simulink model "FCS_MPC_6ph_Regelungsmodell"  (R2022a)
settings: Solver=ode23t  StartTime=0.0  StopTime=0.1  RelTol=1e-3  AbsTol=1e-3  EnableMultiTasking=on
values from neighbouring files (symbols this model uses):
  f_c = 100000    [Params_testbench.m]
  L_d = 0.0001473    [Params_testbench.m]
  L_q = 0.0001484    [Params_testbench.m]
  L_x = 0.00005566    (= 5.566e-05)    [Params_testbench.m]
  L_y = L_x    (= 5.566e-05)    [Params_testbench.m]
  p = 5    [Params_testbench.m]
  psi_pm = 0.0048    [Params_testbench.m]
  R_ph = 0.1278    [Params_testbench.m]
  T_100MHz = 1/f_100MHz    (= 1e-08)    [Params_testbench.m]
  u_dc = 36.0    (= 36)    [Params_testbench.m]
libraries: hdlsllib x53, nesl_utility x39, fl_lib x32, ee_lib x12, simulink x8, spsAlphaBetaZerotodq0Lib x1
(part 5 of 8)

== system FCS_MPC_6ph_Regelungsmodell/Microcontroller Software/Switching_states ==
  I : Inport
  valid_in : Inport  Port=2
  Delay{,1..15} (16 alike) : Delay  DelayLength=1
  Demux : Demux  Outputs=12
  Detect Rise Positive : hdlsllib/Logic and Bit Operations/Detect Rise Positive  vinit=0  OutDataTypeStr=boolean
      settings: SourceProductBaseCode=SL
  MATLAB Function1 : MATLAB Function  TreatAsAtomicUnit=on
  Switch_on2 : Switch  Threshold=1  OutDataTypeStr=Inherit: Inherit via back propagation  RndMeth=Simplest  SaturateOnIntegerOverflow=off  InputSameDT=off
  HB1T : Outport
  HB1B : Outport  Port=2
  HB2T : Outport  Port=3
  HB2B : Outport  Port=4
  HB3T : Outport  Port=5
  HB3B : Outport  Port=6
  HB4T : Outport  Port=7
  HB4B : Outport  Port=8
  HB5T : Outport  Port=9
  HB5B : Outport  Port=10
  HB6T : Outport  Port=11
  HB6B : Outport  Port=12
  done : Outport  Port=13
  wires:
  Demux/4 -> Delay12/1
  I/1 -> Delay1/1
  Demux/6 -> Delay10/1
  Demux/12 -> Delay4/1
  Switch_on2/1 -> MATLAB Function1/1(I), Delay2/1
  Demux/8 -> Delay8/1
  valid_in/1 -> Delay/1
  Demux/7 -> Delay9/1
  Demux/2 -> Delay14/1
  Detect Rise Positive/1 -> Delay3/1, Switch_on2/2  "End_Cycle"
  Demux/5 -> Delay11/1
  Delay2/1 -> Switch_on2/3
  Demux/1 -> Delay15/1
  Demux/9 -> Delay7/1
  Demux/10 -> Delay6/1
  MATLAB Function1/1(next_switching_state) -> Demux/1
  Demux/3 -> Delay13/1
  Delay/1 -> Detect Rise Positive/1
  Delay1/1 -> Switch_on2/1
  Delay3/1 -> done/1
  Delay4/1 -> HB6B/1
  Demux/11 -> Delay5/1
  Delay5/1 -> HB6T/1
  Delay6/1 -> HB5B/1
  Delay7/1 -> HB5T/1
  Delay8/1 -> HB4B/1
  Delay9/1 -> HB4T/1
  Delay10/1 -> HB3B/1
  Delay11/1 -> HB3T/1
  Delay12/1 -> HB2B/1
  Delay13/1 -> HB2T/1
  Delay14/1 -> HB1B/1
  Delay15/1 -> HB1T/1

== system FCS_MPC_6ph_Regelungsmodell/Microcontroller Software/Switching_states1 ==
  I : Inport
  valid_in : Inport  Port=2
  Delay{,1..15} (16 alike) : Delay  DelayLength=1
  Demux : Demux  Outputs=12
  Detect Rise Positive : hdlsllib/Logic and Bit Operations/Detect Rise Positive  vinit=0  OutDataTypeStr=boolean
      settings: SourceProductBaseCode=SL
  MATLAB Function1 : MATLAB Function  TreatAsAtomicUnit=on
  Switch_on2 : Switch  Threshold=1  OutDataTypeStr=Inherit: Inherit via back propagation  RndMeth=Simplest  SaturateOnIntegerOverflow=off  InputSameDT=off
  HB1T : Outport
  HB1B : Outport  Port=2
  HB2T : Outport  Port=3
  HB2B : Outport  Port=4
  HB3T : Outport  Port=5
  HB3B : Outport  Port=6
  HB4T : Outport  Port=7
  HB4B : Outport  Port=8
  HB5T : Outport  Port=9
  HB5B : Outport  Port=10
  HB6T : Outport  Port=11
  HB6B : Outport  Port=12
  done : Outport  Port=13
  wires:
  Demux/4 -> Delay12/1
  I/1 -> Delay1/1
  Demux/6 -> Delay10/1
  Demux/12 -> Delay4/1
  Switch_on2/1 -> MATLAB Function1/1(I), Delay2/1
  Demux/8 -> Delay8/1
  valid_in/1 -> Delay/1
  Demux/7 -> Delay9/1
  Demux/2 -> Delay14/1
  Detect Rise Positive/1 -> Delay3/1, Switch_on2/2  "End_Cycle"
  Demux/5 -> Delay11/1
  Delay2/1 -> Switch_on2/3
  Demux/1 -> Delay15/1
  Demux/9 -> Delay7/1
  Demux/10 -> Delay6/1
  MATLAB Function1/1(next_switching_state) -> Demux/1
  Demux/3 -> Delay13/1
  Delay/1 -> Detect Rise Positive/1
  Delay1/1 -> Switch_on2/1
  Delay3/1 -> done/1
  Delay4/1 -> HB6B/1
  Demux/11 -> Delay5/1
  Delay5/1 -> HB6T/1
  Delay6/1 -> HB5B/1
  Delay7/1 -> HB5T/1
  Delay8/1 -> HB4B/1
  Delay9/1 -> HB4T/1
  Delay10/1 -> HB3B/1
  Delay11/1 -> HB3T/1
  Delay12/1 -> HB2B/1
  Delay13/1 -> HB2T/1
  Delay14/1 -> HB1B/1
  Delay15/1 -> HB1T/1

== system FCS_MPC_6ph_Regelungsmodell/Microcontroller Software/vsd_and_park_tra ==
  i_a1 : Inport
  i_b1 : Inport  Port=2
  i_c1 : Inport  Port=3
  i_a2 : Inport  Port=4
  i_b2 : Inport  Port=5
  i_c2 : Inport  Port=6
  theta_el : Inport  Port=7
  theta_el_offset_ : Inport  Port=8
  curent_valid_in : Inport  Port=9
  Add1 : Sum  Inputs=+-  OutDataTypeStr=Inherit: Same as accumulator  RndMeth=Simplest
  Add2 : Sum  Inputs=-+  RndMeth=Simplest  OutDataTypeStr=Inherit: Same as first input
  Add3 : Sum  RndMeth=Simplest  OutDataTypeStr=Inherit: Same as first input
  Compare To Constant : hdlsllib/Logic and Bit Operations/Compare To Constant  relop=>=  const=2*pi  OutDataTypeStr=boolean
      settings: SourceProductBaseCode=SL
  Compare To Constant1 : hdlsllib/Logic and Bit Operations/Compare To Constant  relop=<  const=0  OutDataTypeStr=boolean
      settings: SourceProductBaseCode=SL
  Constant : Constant  Value=2*pi  OutDataTypeStr=single  SampleTime=1.0000e-08
  Constant1 : Constant  Value=2*pi  OutDataTypeStr=single  SampleTime=1.0000e-08
  Delay{1..6,8,25} (8 alike) : Delay  DelayLength=1
  Detect Rise Positive : hdlsllib/Logic and Bit Operations/Detect Rise Positive  vinit=0  OutDataTypeStr=boolean
      settings: SourceProductBaseCode=SL
  Gain : Gain  Commented=on  Gain=2*pi  OutDataTypeStr=Inherit: Same as input  ParamDataTypeStr=Inherit: Same as input
  MATLAB Function : MATLAB Function  TreatAsAtomicUnit=on
  MATLAB Function1 : MATLAB Function  Commented=on  TreatAsAtomicUnit=on
  Sincos : Trigonometry  Operator=sincos
  Sine HDL Optimized : hdlsllib/Lookup Tables/Cosine HDL Optimized  Commented=on  OutputFormula=sin(2*pi*u) and cos(2*pi*u)  NumDataPoints=512  TableDataTypeStr=fixdt(1,17,11)  SimulateLUTROMDelay=off
      settings: SourceProductBaseCode=SL
  Switch : Switch  Criteria=u2 > Threshold  RndMeth=Simplest  SaturateOnIntegerOverflow=off  InputSameDT=off  OutDataTypeStr=Inherit: Same as first input
  Switch1 : Switch  Criteria=u2 > Threshold  RndMeth=Simplest  SaturateOnIntegerOverflow=off  InputSameDT=off  OutDataTypeStr=Inherit: Same as first input
  Switch_on{1..8} (8 alike) : Switch  Threshold=1  RndMeth=Simplest  SaturateOnIntegerOverflow=off  InputSameDT=off  OutDataTypeStr=Inherit: Same as first input
  i_alpha : Outport
  i_alpha_axi : Outport  Port=2
  i_beta : Outport  Port=3
  i_beta_axi : Outport  Port=4
  i_d : Outport  Port=5
  i_d_axi : Outport  Port=6
  i_q : Outport  Port=7
  i_q_axi : Outport  Port=8
  i_x : Outport  Port=9
  i_x_axi : Outport  Port=10
  i_y : Outport  Port=11
  i_y_axi : Outport  Port=12
  i_0_plus : Outport  Port=13
  i_0_plus_axi : Outport  Port=14
  i_0_minus : Outport  Port=15
  i_0_minus_axi : Outport  Port=16
  done : Outport  Port=17
  i_a1_axi : Outport  Port=18
  i_b1_axi : Outport  Port=19
  i_c1_axi : Outport  Port=20
  i_a2_axi : Outport  Port=21
  i_b2_axi : Outport  Port=22
  i_c2_axi : Outport  Port=23
  theta_test : Outport  Port=24
  wires:
  i_c2/1 -> Switch_on5/1  "End_Cycle"
  Switch_on8/1 -> Add1/1, Delay8/1
  Delay8/1 -> Switch_on8/3
  Detect Rise Positive/1 -> done/1, Switch_on7/2, Switch_on6/2, Switch_on1/2, Switch_on2/2, Switch_on3/2, Switch_on4/2, Switch_on5/2, Switch_on8/2  "End_Cycle"
  Delay4/1 -> Switch_on4/3
  Switch_on2/1 -> Delay2/1, i_c1_axi/1, MATLAB Function/3(i_c1)
  Delay1/1 -> Switch_on1/3
  Switch_on1/1 -> Delay1/1, i_b1_axi/1, MATLAB Function/2(i_b1)
  Switch_on6/1 -> i_a1_axi/1, MATLAB Function/1(i_a1), Delay6/1
  Switch_on4/1 -> Delay4/1, i_b2_axi/1, MATLAB Function/5(i_b2)
  curent_valid_in/1 -> Detect Rise Positive/1  "End_Cycle"
  Switch/1 -> Switch1/3
  Switch_on3/1 -> i_a2_axi/1, MATLAB Function/4(i_a2), Delay3/1
  Delay6/1 -> Switch_on6/3
  Constant/1 -> Add2/1
  Add1/1 -> Switch/3, Compare To Constant1/1, Add3/1, Compare To Constant/1, Add2/2
  Delay2/1 -> Switch_on2/3
  Constant1/1 -> Add3/2
  theta_el/1 -> Switch_on8/1  "End_Cycle"
  Delay3/1 -> Switch_on3/3
  i_a1/1 -> Switch_on6/1  "End_Cycle"
  i_b2/1 -> Switch_on4/1  "End_Cycle"
  Add2/1 -> Switch/1
  i_a2/1 -> Switch_on3/1  "End_Cycle"
  i_b1/1 -> Switch_on1/1  "End_Cycle"
  Delay5/1 -> Switch_on5/3
  Add3/1 -> Switch1/1
  i_c1/1 -> Switch_on2/1  "End_Cycle"
  MATLAB Function/1(i_alpha) -> i_alpha_axi/1, i_alpha/1  "curent_valid_in"
  MATLAB Function/2(i_beta) -> i_beta_axi/1, i_beta/1  "curent_valid_in"
  MATLAB Function/3(i_x) -> i_x_axi/1, i_x/1  "curent_valid_in"
  Compare To Constant/1 -> Switch/2
  Compare To Constant1/1 -> Switch1/2
  Switch_on7/1 -> Add1/2, Delay25/1
  Delay25/1 -> Switch_on7/3
  Switch1/1 -> Sincos/1  "End_Cycle"
  ? -> Sine HDL Optimized/1
  theta_el_offset_/1 -> Switch_on7/1
  MATLAB Function/8(i_q) -> i_q_axi/1, i_q/1
  MATLAB Function/7(i_d) -> i_d_axi/1, i_d/1
  MATLAB Function/6(i_0_minus) -> i_0_minus_axi/1, i_0_minus/1
  MATLAB Function/5(i_0_plus) -> i_0_plus_axi/1, i_0_plus/1
  MATLAB Function/4(i_y) -> i_y_axi/1, i_y/1
  Switch_on5/1 -> Delay5/1, i_c2_axi/1, MATLAB Function/6(i_c2)
  Sincos/1 -> MATLAB Function/7(sin_theta_el)
  Sincos/2 -> theta_test/1, MATLAB Function/8(cos_theta_el)

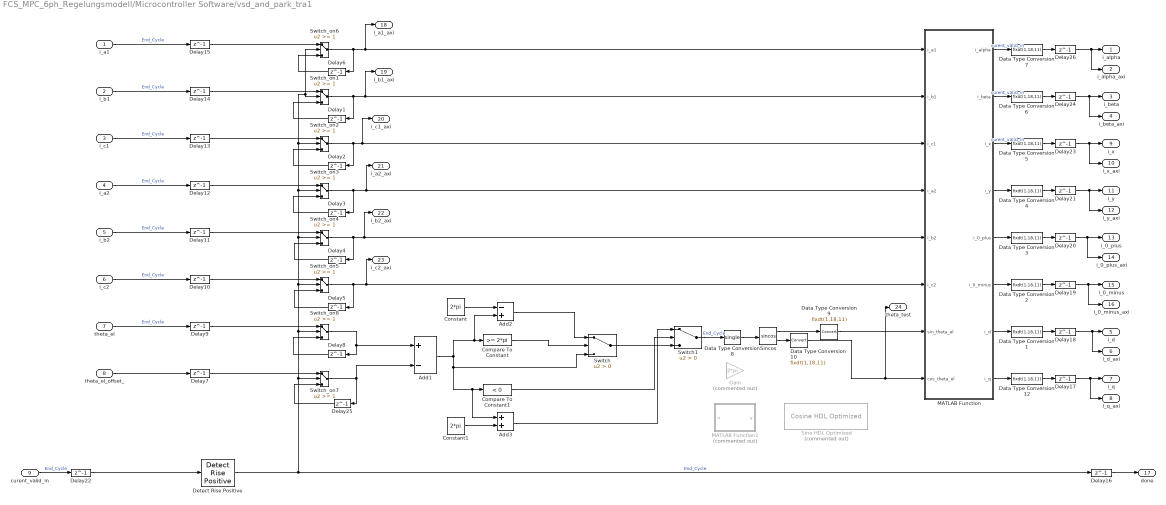
== system FCS_MPC_6ph_Regelungsmodell/Microcontroller Software/vsd_and_park_tra1 ==
  i_a1 : Inport
  i_b1 : Inport  Port=2
  i_c1 : Inport  Port=3
  i_a2 : Inport  Port=4
  i_b2 : Inport  Port=5
  i_c2 : Inport  Port=6
  theta_el : Inport  Port=7
  theta_el_offset_ : Inport  Port=8
  curent_valid_in : Inport  Port=9
  Add1 : Sum  Inputs=+-  OutDataTypeStr=Inherit: Same as accumulator  RndMeth=Simplest
  Add2 : Sum  Inputs=-+  RndMeth=Simplest
  Add3 : Sum  RndMeth=Simplest  OutDataTypeStr=Inherit: Same as first input
  Compare To Constant : hdlsllib/Logic and Bit Operations/Compare To Constant  relop=>=  const=2*pi  OutDataTypeStr=boolean
      settings: SourceProductBaseCode=SL
  Compare To Constant1 : hdlsllib/Logic and Bit Operations/Compare To Constant  relop=<  const=0  OutDataTypeStr=boolean
      settings: SourceProductBaseCode=SL
  Constant : Constant  Value=2*pi  OutDataTypeStr=fixdt(1,24,20)  SampleTime=1.0000e-08
  Constant1 : Constant  Value=2*pi  OutDataTypeStr=fixdt(1,24,20)  SampleTime=1.0000e-08
  Data Type Conversion{1..7,9..10,12} (10 alike) : DataTypeConversion  OutDataTypeStr=fixdt(1,18,11)  RndMeth=Simplest  SaturateOnIntegerOverflow=off
  Data Type Conversion8 : DataTypeConversion  OutDataTypeStr=single  RndMeth=Simplest  SaturateOnIntegerOverflow=off
  Delay{1..26} (26 alike) : Delay  DelayLength=1
  Detect Rise Positive : hdlsllib/Logic and Bit Operations/Detect Rise Positive  vinit=0  OutDataTypeStr=boolean
      settings: SourceProductBaseCode=SL
  Gain : Gain  Commented=on  Gain=2*pi  OutDataTypeStr=Inherit: Same as input  ParamDataTypeStr=Inherit: Same as input
  MATLAB Function : MATLAB Function  TreatAsAtomicUnit=on
  MATLAB Function1 : MATLAB Function  Commented=on  TreatAsAtomicUnit=on
  Sincos : Trigonometry  Operator=sincos
  Sine HDL Optimized : hdlsllib/Lookup Tables/Cosine HDL Optimized  Commented=on  OutputFormula=sin(2*pi*u) and cos(2*pi*u)  NumDataPoints=512  TableDataTypeStr=fixdt(1,17,11)  SimulateLUTROMDelay=off
      settings: SourceProductBaseCode=SL
  Switch : Switch  Criteria=u2 > Threshold  OutDataTypeStr=fixdt(1,24,20)  RndMeth=Simplest  SaturateOnIntegerOverflow=off  InputSameDT=off
  Switch1 : Switch  Criteria=u2 > Threshold  OutDataTypeStr=fixdt(1,24,20)  RndMeth=Simplest  SaturateOnIntegerOverflow=off  InputSameDT=off
  Switch_on{1..8} (8 alike) : Switch  Threshold=1  RndMeth=Simplest  SaturateOnIntegerOverflow=off  InputSameDT=off  OutDataTypeStr=Inherit: Same as first input
  i_alpha : Outport
  i_alpha_axi : Outport  Port=2
  i_beta : Outport  Port=3
  i_beta_axi : Outport  Port=4
  i_d : Outport  Port=5
  i_d_axi : Outport  Port=6
  i_q : Outport  Port=7
  i_q_axi : Outport  Port=8
  i_x : Outport  Port=9
  i_x_axi : Outport  Port=10
  i_y : Outport  Port=11
  i_y_axi : Outport  Port=12
  i_0_plus : Outport  Port=13
  i_0_plus_axi : Outport  Port=14
  i_0_minus : Outport  Port=15
  i_0_minus_axi : Outport  Port=16
  done : Outport  Port=17
  i_a1_axi : Outport  Port=18
  i_b1_axi : Outport  Port=19
  i_c1_axi : Outport  Port=20
  i_a2_axi : Outport  Port=21
  i_b2_axi : Outport  Port=22
  i_c2_axi : Outport  Port=23
  theta_test : Outport  Port=24
  wires:
  i_c2/1 -> Delay10/1  "End_Cycle"
  Switch_on8/1 -> Add1/1, Delay8/1
  Delay8/1 -> Switch_on8/3
  Detect Rise Positive/1 -> Delay16/1, Switch_on7/2, Switch_on6/2, Switch_on1/2, Switch_on2/2, Switch_on3/2, Switch_on4/2, Switch_on5/2, Switch_on8/2  "End_Cycle"
  Delay4/1 -> Switch_on4/3
  Switch_on2/1 -> Delay2/1, i_c1_axi/1, MATLAB Function/3(i_c1)
  Delay1/1 -> Switch_on1/3
  Switch_on1/1 -> Delay1/1, i_b1_axi/1, MATLAB Function/2(i_b1)
  Switch_on6/1 -> i_a1_axi/1, MATLAB Function/1(i_a1), Delay6/1
  Switch_on4/1 -> Delay4/1, i_b2_axi/1, MATLAB Function/5(i_b2)
  curent_valid_in/1 -> Delay22/1  "End_Cycle"
  Switch/1 -> Switch1/3
  Switch_on3/1 -> i_a2_axi/1, MATLAB Function/4(i_a2), Delay3/1
  Delay6/1 -> Switch_on6/3
  Constant/1 -> Add2/1
  Add1/1 -> Switch/3, Compare To Constant1/1, Add3/1, Compare To Constant/1, Add2/2
  Delay2/1 -> Switch_on2/3
  Constant1/1 -> Add3/2
  theta_el/1 -> Delay9/1  "End_Cycle"
  Delay3/1 -> Switch_on3/3
  i_a1/1 -> Delay15/1  "End_Cycle"
  i_b2/1 -> Delay11/1  "End_Cycle"
  Add2/1 -> Switch/1
  i_a2/1 -> Delay12/1  "End_Cycle"
  i_b1/1 -> Delay14/1  "End_Cycle"
  Delay5/1 -> Switch_on5/3
  Add3/1 -> Switch1/1
  i_c1/1 -> Delay13/1  "End_Cycle"
  MATLAB Function/4(i_y) -> Data Type Conversion4/1
  MATLAB Function/5(i_0_plus) -> Data Type Conversion3/1
  MATLAB Function/6(i_0_minus) -> Data Type Conversion2/1
  MATLAB Function/7(i_d) -> Data Type Conversion1/1
  MATLAB Function/8(i_q) -> Data Type Conversion12/1
  MATLAB Function/1(i_alpha) -> Data Type Conversion7/1  "curent_valid_in"
  MATLAB Function/2(i_beta) -> Data Type Conversion6/1  "curent_valid_in"
  MATLAB Function/3(i_x) -> Data Type Conversion5/1  "curent_valid_in"
  Data Type Conversion12/1 -> Delay17/1
  Data Type Conversion1/1 -> Delay18/1
  Data Type Conversion2/1 -> Delay19/1
  Data Type Conversion3/1 -> Delay20/1
  Data Type Conversion4/1 -> Delay21/1
  Data Type Conversion5/1 -> Delay23/1
  Data Type Conversion6/1 -> Delay24/1
  Data Type Conversion7/1 -> Delay26/1
  Compare To Constant/1 -> Switch/2
  Compare To Constant1/1 -> Switch1/2
  Switch_on7/1 -> Add1/2, Delay25/1
  Delay25/1 -> Switch_on7/3
  Sincos/1 -> Data Type Conversion9/1
  Sincos/2 -> Data Type Conversion10/1
  theta_el_offset_/1 -> Delay7/1
  Switch1/1 -> Data Type Conversion8/1  "End_Cycle"
  ? -> Sine HDL Optimized/1
  Delay22/1 -> Detect Rise Positive/1
  Delay7/1 -> Switch_on7/1
  Delay9/1 -> Switch_on8/1
  Delay10/1 -> Switch_on5/1
  Delay11/1 -> Switch_on4/1
  Delay12/1 -> Switch_on3/1
  Delay13/1 -> Switch_on2/1
  Delay14/1 -> Switch_on1/1
  Delay15/1 -> Switch_on6/1
  Delay16/1 -> done/1
  Delay17/1 -> i_q_axi/1, i_q/1
  Delay18/1 -> i_d_axi/1, i_d/1
  Delay19/1 -> i_0_minus_axi/1, i_0_minus/1
  Delay20/1 -> i_0_plus_axi/1, i_0_plus/1
  Delay21/1 -> i_y_axi/1, i_y/1
  Delay23/1 -> i_x_axi/1, i_x/1
  Delay24/1 -> i_beta_axi/1, i_beta/1
  Delay26/1 -> i_alpha_axi/1, i_alpha/1
  Switch_on5/1 -> Delay5/1, i_c2_axi/1, MATLAB Function/6(i_c2)
  Data Type Conversion8/1 -> Sincos/1
  Data Type Conversion9/1 -> MATLAB Function/7(sin_theta_el)
  Data Type Conversion10/1 -> theta_test/1, MATLAB Function/8(cos_theta_el)

== system FCS_MPC_6ph_Regelungsmodell/Microcontroller Software/Phase_voltages_per_switching_state1/Subsystem ==
  u_dc_link_voltage15 : Inport
  Index 15 : Inport  Port=2
  sin_theta_el : Inport  Port=3
  cos_theta_el : Inport  Port=4
  MATLAB Function10 : MATLAB Function  TreatAsAtomicUnit=on
  MATLAB Function11 : MATLAB Function  TreatAsAtomicUnit=on
  MATLAB Function12 : MATLAB Function  TreatAsAtomicUnit=on
  MATLAB Function13 : MATLAB Function  TreatAsAtomicUnit=on
  MATLAB Function14 : MATLAB Function  TreatAsAtomicUnit=on
  MATLAB Function15 : MATLAB Function  TreatAsAtomicUnit=on
  MATLAB Function8 : MATLAB Function  TreatAsAtomicUnit=on
  MATLAB Function9 : MATLAB Function  TreatAsAtomicUnit=on
  d_voltage_per_switching_state : Outport
  q_voltage_per_switching_state : Outport  Port=2
  x_voltage_per_switching_state : Outport  Port=3
  y_voltage_per_switching_state : Outport  Port=4
  d_voltage_per_switching_state1 : Outport  Port=5
  q_voltage_per_switching_state1 : Outport  Port=6
  x_voltage_per_switching_state1 : Outport  Port=7
  y_voltage_per_switching_state1 : Outport  Port=8
  d_voltage_per_switching_state2 : Outport  Port=9
  q_voltage_per_switching_state2 : Outport  Port=10
  x_voltage_per_switching_state2 : Outport  Port=11
  y_voltage_per_switching_state2 : Outport  Port=12
  d_voltage_per_switching_state3 : Outport  Port=13
  q_voltage_per_switching_state3 : Outport  Port=14
  x_voltage_per_switching_state3 : Outport  Port=15
  y_voltage_per_switching_state3 : Outport  Port=16
  d_voltage_per_switching_state4 : Outport  Port=17
  q_voltage_per_switching_state4 : Outport  Port=18
  x_voltage_per_switching_state4 : Outport  Port=19
  y_voltage_per_switching_state4 : Outport  Port=20
  d_voltage_per_switching_state5 : Outport  Port=21
  q_voltage_per_switching_state5 : Outport  Port=22
  x_voltage_per_switching_state5 : Outport  Port=23
  y_voltage_per_switching_state5 : Outport  Port=24
  d_voltage_per_switching_state6 : Outport  Port=25
  q_voltage_per_switching_state6 : Outport  Port=26
  x_voltage_per_switching_state6 : Outport  Port=27
  y_voltage_per_switching_state6 : Outport  Port=28
  d_voltage_per_switching_state7 : Outport  Port=29
  q_voltage_per_switching_state7 : Outport  Port=30
  x_voltage_per_switching_state7 : Outport  Port=31
  y_voltage_per_switching_state7 : Outport  Port=32
  wires:
  MATLAB Function11/4(y_voltage_per_switching_state) -> y_voltage_per_switching_state4/1
  MATLAB Function10/3(x_voltage_per_switching_state) -> x_voltage_per_switching_state5/1
  MATLAB Function8/1(d_voltage_per_switching_state) -> d_voltage_per_switching_state7/1
  MATLAB Function8/2(q_voltage_per_switching_state) -> q_voltage_per_switching_state7/1
  MATLAB Function11/1(d_voltage_per_switching_state) -> d_voltage_per_switching_state4/1
  MATLAB Function12/3(x_voltage_per_switching_state) -> x_voltage_per_switching_state3/1
  MATLAB Function15/2(q_voltage_per_switching_state) -> q_voltage_per_switching_state/1
  MATLAB Function8/3(x_voltage_per_switching_state) -> x_voltage_per_switching_state7/1
  MATLAB Function11/3(x_voltage_per_switching_state) -> x_voltage_per_switching_state4/1
  MATLAB Function10/4(y_voltage_per_switching_state) -> y_voltage_per_switching_state5/1
  MATLAB Function11/2(q_voltage_per_switching_state) -> q_voltage_per_switching_state4/1
  MATLAB Function12/1(d_voltage_per_switching_state) -> d_voltage_per_switching_state3/1
  MATLAB Function12/4(y_voltage_per_switching_state) -> y_voltage_per_switching_state3/1
  MATLAB Function13/2(q_voltage_per_switching_state) -> q_voltage_per_switching_state2/1
  MATLAB Function10/1(d_voltage_per_switching_state) -> d_voltage_per_switching_state5/1
  MATLAB Function10/2(q_voltage_per_switching_state) -> q_voltage_per_switching_state5/1
  MATLAB Function13/4(y_voltage_per_switching_state) -> y_voltage_per_switching_state2/1
  MATLAB Function8/4(y_voltage_per_switching_state) -> y_voltage_per_switching_state7/1
  MATLAB Function13/1(d_voltage_per_switching_state) -> d_voltage_per_switching_state2/1
  MATLAB Function13/3(x_voltage_per_switching_state) -> x_voltage_per_switching_state2/1
  MATLAB Function12/2(q_voltage_per_switching_state) -> q_voltage_per_switching_state3/1
  MATLAB Function15/1(d_voltage_per_switching_state) -> d_voltage_per_switching_state/1
  MATLAB Function15/4(y_voltage_per_switching_state) -> y_voltage_per_switching_state/1
  MATLAB Function15/3(x_voltage_per_switching_state) -> x_voltage_per_switching_state/1
  u_dc_link_voltage15/1 -> MATLAB Function8/3(u_dc_link_voltage), MATLAB Function9/3(u_dc_link_voltage), MATLAB Function10/3(u_dc_link_voltage), MATLAB Function11/3(u_dc_link_voltage), MATLAB Function12/3(u_dc_link_voltage), MATLAB Function13/3(u_dc_link_voltage), MATLAB Function14/3(u_dc_link_voltage), MATLAB Function15/3(u_dc_link_voltage)
  MATLAB Function14/4(y_voltage_per_switching_state) -> y_voltage_per_switching_state1/1
  MATLAB Function14/3(x_voltage_per_switching_state) -> x_voltage_per_switching_state1/1
  MATLAB Function14/1(d_voltage_per_switching_state) -> d_voltage_per_switching_state1/1
  MATLAB Function14/2(q_voltage_per_switching_state) -> q_voltage_per_switching_state1/1
  Index 15/1 -> MATLAB Function15/4(Index), MATLAB Function10/4(Index), MATLAB Function8/4(Index), MATLAB Function9/4(Index), MATLAB Function11/4(Index), MATLAB Function12/4(Index), MATLAB Function13/4(Index), MATLAB Function14/4(Index)
  MATLAB Function9/3(x_voltage_per_switching_state) -> x_voltage_per_switching_state6/1
  MATLAB Function9/2(q_voltage_per_switching_state) -> q_voltage_per_switching_state6/1
  MATLAB Function9/1(d_voltage_per_switching_state) -> d_voltage_per_switching_state6/1
  MATLAB Function9/4(y_voltage_per_switching_state) -> y_voltage_per_switching_state6/1
  sin_theta_el/1 -> MATLAB Function14/1(sin_theta_el), MATLAB Function8/1(sin_theta_el), MATLAB Function9/1(sin_theta_el), MATLAB Function10/1(sin_theta_el), MATLAB Function11/1(sin_theta_el), MATLAB Function12/1(sin_theta_el), MATLAB Function13/1(sin_theta_el), MATLAB Function15/1(sin_theta_el)
  cos_theta_el/1 -> MATLAB Function15/2(cos_theta_el), MATLAB Function8/2(cos_theta_el), MATLAB Function9/2(cos_theta_el), MATLAB Function10/2(cos_theta_el), MATLAB Function11/2(cos_theta_el), MATLAB Function12/2(cos_theta_el), MATLAB Function13/2(cos_theta_el), MATLAB Function14/2(cos_theta_el)

== system FCS_MPC_6ph_Regelungsmodell/Microcontroller Software/Phase_voltages_per_switching_state2/Subsystem ==
  u_dc_link_voltage15 : Inport
  Index 15 : Inport  Port=2
  sin_theta_el : Inport  Port=3
  cos_theta_el : Inport  Port=4
  MATLAB Function10 : MATLAB Function  TreatAsAtomicUnit=on
  MATLAB Function11 : MATLAB Function  TreatAsAtomicUnit=on
  MATLAB Function12 : MATLAB Function  TreatAsAtomicUnit=on
  MATLAB Function13 : MATLAB Function  TreatAsAtomicUnit=on
  MATLAB Function14 : MATLAB Function  TreatAsAtomicUnit=on
  MATLAB Function15 : MATLAB Function  TreatAsAtomicUnit=on
  MATLAB Function8 : MATLAB Function  TreatAsAtomicUnit=on
  MATLAB Function9 : MATLAB Function  TreatAsAtomicUnit=on
  d_voltage_per_switching_state : Outport
  q_voltage_per_switching_state : Outport  Port=2
  x_voltage_per_switching_state : Outport  Port=3
  y_voltage_per_switching_state : Outport  Port=4
  d_voltage_per_switching_state1 : Outport  Port=5
  q_voltage_per_switching_state1 : Outport  Port=6
  x_voltage_per_switching_state1 : Outport  Port=7
  y_voltage_per_switching_state1 : Outport  Port=8
  d_voltage_per_switching_state2 : Outport  Port=9
  q_voltage_per_switching_state2 : Outport  Port=10
  x_voltage_per_switching_state2 : Outport  Port=11
  y_voltage_per_switching_state2 : Outport  Port=12
  d_voltage_per_switching_state3 : Outport  Port=13
  q_voltage_per_switching_state3 : Outport  Port=14
  x_voltage_per_switching_state3 : Outport  Port=15
  y_voltage_per_switching_state3 : Outport  Port=16
  d_voltage_per_switching_state4 : Outport  Port=17
  q_voltage_per_switching_state4 : Outport  Port=18
  x_voltage_per_switching_state4 : Outport  Port=19
  y_voltage_per_switching_state4 : Outport  Port=20
  d_voltage_per_switching_state5 : Outport  Port=21
  q_voltage_per_switching_state5 : Outport  Port=22
  x_voltage_per_switching_state5 : Outport  Port=23
  y_voltage_per_switching_state5 : Outport  Port=24
  d_voltage_per_switching_state6 : Outport  Port=25
  q_voltage_per_switching_state6 : Outport  Port=26
  x_voltage_per_switching_state6 : Outport  Port=27
  y_voltage_per_switching_state6 : Outport  Port=28
  d_voltage_per_switching_state7 : Outport  Port=29
  q_voltage_per_switching_state7 : Outport  Port=30
  x_voltage_per_switching_state7 : Outport  Port=31
  y_voltage_per_switching_state7 : Outport  Port=32
  wires:
  MATLAB Function11/4(y_voltage_per_switching_state) -> y_voltage_per_switching_state4/1
  MATLAB Function10/3(x_voltage_per_switching_state) -> x_voltage_per_switching_state5/1
  MATLAB Function8/1(d_voltage_per_switching_state) -> d_voltage_per_switching_state7/1
  MATLAB Function8/2(q_voltage_per_switching_state) -> q_voltage_per_switching_state7/1
  MATLAB Function11/1(d_voltage_per_switching_state) -> d_voltage_per_switching_state4/1
  MATLAB Function12/3(x_voltage_per_switching_state) -> x_voltage_per_switching_state3/1
  MATLAB Function15/2(q_voltage_per_switching_state) -> q_voltage_per_switching_state/1
  MATLAB Function8/3(x_voltage_per_switching_state) -> x_voltage_per_switching_state7/1
  MATLAB Function11/3(x_voltage_per_switching_state) -> x_voltage_per_switching_state4/1
  MATLAB Function10/4(y_voltage_per_switching_state) -> y_voltage_per_switching_state5/1
  MATLAB Function11/2(q_voltage_per_switching_state) -> q_voltage_per_switching_state4/1
  MATLAB Function12/1(d_voltage_per_switching_state) -> d_voltage_per_switching_state3/1
  MATLAB Function12/4(y_voltage_per_switching_state) -> y_voltage_per_switching_state3/1
  MATLAB Function13/2(q_voltage_per_switching_state) -> q_voltage_per_switching_state2/1
  MATLAB Function10/1(d_voltage_per_switching_state) -> d_voltage_per_switching_state5/1
  MATLAB Function10/2(q_voltage_per_switching_state) -> q_voltage_per_switching_state5/1
  MATLAB Function13/4(y_voltage_per_switching_state) -> y_voltage_per_switching_state2/1
  MATLAB Function8/4(y_voltage_per_switching_state) -> y_voltage_per_switching_state7/1
  MATLAB Function13/1(d_voltage_per_switching_state) -> d_voltage_per_switching_state2/1
  MATLAB Function13/3(x_voltage_per_switching_state) -> x_voltage_per_switching_state2/1
  MATLAB Function12/2(q_voltage_per_switching_state) -> q_voltage_per_switching_state3/1
  MATLAB Function15/1(d_voltage_per_switching_state) -> d_voltage_per_switching_state/1
  MATLAB Function15/4(y_voltage_per_switching_state) -> y_voltage_per_switching_state/1
  MATLAB Function15/3(x_voltage_per_switching_state) -> x_voltage_per_switching_state/1
  u_dc_link_voltage15/1 -> MATLAB Function8/3(u_dc_link_voltage), MATLAB Function9/3(u_dc_link_voltage), MATLAB Function10/3(u_dc_link_voltage), MATLAB Function11/3(u_dc_link_voltage), MATLAB Function12/3(u_dc_link_voltage), MATLAB Function13/3(u_dc_link_voltage), MATLAB Function14/3(u_dc_link_voltage), MATLAB Function15/3(u_dc_link_voltage)
  MATLAB Function14/4(y_voltage_per_switching_state) -> y_voltage_per_switching_state1/1
  MATLAB Function14/3(x_voltage_per_switching_state) -> x_voltage_per_switching_state1/1
  MATLAB Function14/1(d_voltage_per_switching_state) -> d_voltage_per_switching_state1/1
  MATLAB Function14/2(q_voltage_per_switching_state) -> q_voltage_per_switching_state1/1
  Index 15/1 -> MATLAB Function15/4(Index), MATLAB Function10/4(Index), MATLAB Function8/4(Index), MATLAB Function9/4(Index), MATLAB Function11/4(Index), MATLAB Function12/4(Index), MATLAB Function13/4(Index), MATLAB Function14/4(Index)
  MATLAB Function9/3(x_voltage_per_switching_state) -> x_voltage_per_switching_state6/1
  MATLAB Function9/2(q_voltage_per_switching_state) -> q_voltage_per_switching_state6/1
  MATLAB Function9/1(d_voltage_per_switching_state) -> d_voltage_per_switching_state6/1
  MATLAB Function9/4(y_voltage_per_switching_state) -> y_voltage_per_switching_state6/1
  sin_theta_el/1 -> MATLAB Function14/1(sin_theta_el), MATLAB Function8/1(sin_theta_el), MATLAB Function9/1(sin_theta_el), MATLAB Function10/1(sin_theta_el), MATLAB Function11/1(sin_theta_el), MATLAB Function12/1(sin_theta_el), MATLAB Function13/1(sin_theta_el), MATLAB Function15/1(sin_theta_el)
  cos_theta_el/1 -> MATLAB Function15/2(cos_theta_el), MATLAB Function8/2(cos_theta_el), MATLAB Function9/2(cos_theta_el), MATLAB Function10/2(cos_theta_el), MATLAB Function11/2(cos_theta_el), MATLAB Function12/2(cos_theta_el), MATLAB Function13/2(cos_theta_el), MATLAB Function14/2(cos_theta_el)

== system FCS_MPC_6ph_Regelungsmodell/Microcontroller Software/Prediction_and_cost_function/Subsystem ==
  d_phase_voltage_per_switching_state : Inport
  q_phase_voltage_per_switching_state : Inport  Port=2
  x_phase_voltage_per_switching_state : Inport  Port=3
  y_phase_voltage_per_switching_state : Inport  Port=4
  d_phase_voltage_per_switching_state1 : Inport  Port=5
  q_phase_voltage_per_switching_state1 : Inport  Port=6
  x_phase_voltage_per_switching_state1 : Inport  Port=7
  y_phase_voltage_per_switching_state1 : Inport  Port=8
  d_phase_voltage_per_switching_state2 : Inport  Port=9
  q_phase_voltage_per_switching_state2 : Inport  Port=10
  x_phase_voltage_per_switching_state2 : Inport  Port=11
  y_phase_voltage_per_switching_state2 : Inport  Port=12
  d_phase_voltage_per_switching_state3 : Inport  Port=13
  q_phase_voltage_per_switching_state3 : Inport  Port=14
  x_phase_voltage_per_switching_state3 : Inport  Port=15
  y_phase_voltage_per_switching_state3 : Inport  Port=16
  d_phase_voltage_per_switching_state4 : Inport  Port=17
  q_phase_voltage_per_switching_state4 : Inport  Port=18
  x_phase_voltage_per_switching_state4 : Inport  Port=19
  y_phase_voltage_per_switching_state4 : Inport  Port=20
  d_phase_voltage_per_switching_state5 : Inport  Port=21
  q_phase_voltage_per_switching_state5 : Inport  Port=22
  x_phase_voltage_per_switching_state5 : Inport  Port=23
  y_phase_voltage_per_switching_state5 : Inport  Port=24
  d_phase_voltage_per_switching_state6 : Inport  Port=25
  q_phase_voltage_per_switching_state6 : Inport  Port=26
  x_phase_voltage_per_switching_state6 : Inport  Port=27
  y_phase_voltage_per_switching_state6 : Inport  Port=28
  d_phase_voltage_per_switching_state7 : Inport  Port=29
  q_phase_voltage_per_switching_state7 : Inport  Port=30
  x_phase_voltage_per_switching_state7 : Inport  Port=31
  y_phase_voltage_per_switching_state7 : Inport  Port=32
  SampleTime_div_Ld15 : Inport  Port=33
  SampleTime_div_Lq15 : Inport  Port=34
  SampleTime_div_Lx15 : Inport  Port=35
  SampleTime_div_Ly15 : Inport  Port=36
  id_k_16 : Inport  Port=37
  iq_k_16 : Inport  Port=38
  ix_k_16 : Inport  Port=39
  iy_k_16 : Inport  Port=40
  Rs15 : Inport  Port=41
  omega_el15 : Inport  Port=42
  Lq15 : Inport  Port=43
  Ld15 : Inport  Port=44
  psiPM15 : Inport  Port=45
  id_ref15 : Inport  Port=46
  iq_ref15 : Inport  Port=47
  ix_ref15 : Inport  Port=48
  iy_ref15 : Inport  Port=49
  MATLAB Function10 : MATLAB Function  TreatAsAtomicUnit=on
  MATLAB Function11 : MATLAB Function  TreatAsAtomicUnit=on
  MATLAB Function12 : MATLAB Function  TreatAsAtomicUnit=on
  MATLAB Function13 : MATLAB Function  TreatAsAtomicUnit=on
  MATLAB Function14 : MATLAB Function  TreatAsAtomicUnit=on
  MATLAB Function15 : MATLAB Function  TreatAsAtomicUnit=on
  MATLAB Function8 : MATLAB Function  TreatAsAtomicUnit=on
  MATLAB Function9 : MATLAB Function  TreatAsAtomicUnit=on
  J : Outport
  J1 : Outport  Port=2
  J2 : Outport  Port=3
  J3 : Outport  Port=4
  J4 : Outport  Port=5
  J5 : Outport  Port=6
  J6 : Outport  Port=7
  J7 : Outport  Port=8
  wires:
  q_phase_voltage_per_switching_state1/1 -> MATLAB Function14/15(q_phase_voltage_per_switching_state)
  SampleTime_div_Ld15/1 -> MATLAB Function8/1(SampleTime_div_Ld), MATLAB Function9/1(SampleTime_div_Ld), MATLAB Function10/1(SampleTime_div_Ld), MATLAB Function11/1(SampleTime_div_Ld), MATLAB Function12/1(SampleTime_div_Ld), MATLAB Function13/1(SampleTime_div_Ld), MATLAB Function14/1(SampleTime_div_Ld), MATLAB Function15/1(SampleTime_div_Ld)
  Rs15/1 -> MATLAB Function8/9(Rs), MATLAB Function9/9(Rs), MATLAB Function10/9(Rs), MATLAB Function11/9(Rs), MATLAB Function12/9(Rs), MATLAB Function13/9(Rs), MATLAB Function14/9(Rs), MATLAB Function15/9(Rs)
  y_phase_voltage_per_switching_state/1 -> MATLAB Function15/17(y_phase_voltage_per_switching_state)
  Lq15/1 -> MATLAB Function8/11(Lq), MATLAB Function9/11(Lq), MATLAB Function10/11(Lq), MATLAB Function11/11(Lq), MATLAB Function12/11(Lq), MATLAB Function13/11(Lq), MATLAB Function14/11(Lq), MATLAB Function15/11(Lq)
  MATLAB Function11/1(J) -> J4/1
  y_phase_voltage_per_switching_state2/1 -> MATLAB Function13/17(y_phase_voltage_per_switching_state)
  d_phase_voltage_per_switching_state1/1 -> MATLAB Function14/14(d_phase_voltage_per_switching_state)
  x_phase_voltage_per_switching_state1/1 -> MATLAB Function14/16(x_phase_voltage_per_switching_state)
  y_phase_voltage_per_switching_state7/1 -> MATLAB Function8/17(y_phase_voltage_per_switching_state)
  iy_ref15/1 -> MATLAB Function8/21(iy_ref), MATLAB Function9/21(iy_ref), MATLAB Function10/21(iy_ref), MATLAB Function11/21(iy_ref), MATLAB Function12/21(iy_ref), MATLAB Function13/21(iy_ref), MATLAB Function14/21(iy_ref), MATLAB Function15/21(iy_ref)
  omega_el15/1 -> MATLAB Function8/10(omega_el), MATLAB Function9/10(omega_el), MATLAB Function10/10(omega_el), MATLAB Function11/10(omega_el), MATLAB Function12/10(omega_el), MATLAB Function13/10(omega_el), MATLAB Function14/10(omega_el), MATLAB Function15/10(omega_el)
  psiPM15/1 -> MATLAB Function8/13(psiPM), MATLAB Function9/13(psiPM), MATLAB Function10/13(psiPM), MATLAB Function11/13(psiPM), MATLAB Function12/13(psiPM), MATLAB Function13/13(psiPM), MATLAB Function14/13(psiPM), MATLAB Function15/13(psiPM)
  d_phase_voltage_per_switching_state3/1 -> MATLAB Function12/14(d_phase_voltage_per_switching_state)
  d_phase_voltage_per_switching_state6/1 -> MATLAB Function9/14(d_phase_voltage_per_switching_state)
  d_phase_voltage_per_switching_state/1 -> MATLAB Function15/14(d_phase_voltage_per_switching_state)
  x_phase_voltage_per_switching_state3/1 -> MATLAB Function12/16(x_phase_voltage_per_switching_state)
  d_phase_voltage_per_switching_state2/1 -> MATLAB Function13/14(d_phase_voltage_per_switching_state)
  x_phase_voltage_per_switching_state4/1 -> MATLAB Function11/16(x_phase_voltage_per_switching_state)
  y_phase_voltage_per_switching_state1/1 -> MATLAB Function14/17(y_phase_voltage_per_switching_state)
  MATLAB Function14/1(J) -> J1/1
  MATLAB Function8/1(J) -> J7/1
  q_phase_voltage_per_switching_state2/1 -> MATLAB Function13/15(q_phase_voltage_per_switching_state)
  x_phase_voltage_per_switching_state2/1 -> MATLAB Function13/16(x_phase_voltage_per_switching_state)
  MATLAB Function13/1(J) -> J2/1
  y_phase_voltage_per_switching_state4/1 -> MATLAB Function11/17(y_phase_voltage_per_switching_state)
  x_phase_voltage_per_switching_state/1 -> MATLAB Function15/16(x_phase_voltage_per_switching_state)
  q_phase_voltage_per_switching_state5/1 -> MATLAB Function10/15(q_phase_voltage_per_switching_state)
  d_phase_voltage_per_switching_state7/1 -> MATLAB Function8/14(d_phase_voltage_per_switching_state)
  d_phase_voltage_per_switching_state4/1 -> MATLAB Function11/14(d_phase_voltage_per_switching_state)
  q_phase_voltage_per_switching_state4/1 -> MATLAB Function11/15(q_phase_voltage_per_switching_state)
  x_phase_voltage_per_switching_state5/1 -> MATLAB Function10/16(x_phase_voltage_per_switching_state)
  SampleTime_div_Lx15/1 -> MATLAB Function8/3(SampleTime_div_Lx), MATLAB Function9/3(SampleTime_div_Lx), MATLAB Function10/3(SampleTime_div_Lx), MATLAB Function11/3(SampleTime_div_Lx), MATLAB Function12/3(SampleTime_div_Lx), MATLAB Function13/3(SampleTime_div_Lx), MATLAB Function14/3(SampleTime_div_Lx), MATLAB Function15/3(SampleTime_div_Lx)
  SampleTime_div_Ly15/1 -> MATLAB Function8/4(SampleTime_div_Ly), MATLAB Function9/4(SampleTime_div_Ly), MATLAB Function10/4(SampleTime_div_Ly), MATLAB Function11/4(SampleTime_div_Ly), MATLAB Function12/4(SampleTime_div_Ly), MATLAB Function13/4(SampleTime_div_Ly), MATLAB Function14/4(SampleTime_div_Ly), MATLAB Function15/4(SampleTime_div_Ly)
  SampleTime_div_Lq15/1 -> MATLAB Function8/2(SampleTime_div_Lq), MATLAB Function9/2(SampleTime_div_Lq), MATLAB Function10/2(SampleTime_div_Lq), MATLAB Function11/2(SampleTime_div_Lq), MATLAB Function12/2(SampleTime_div_Lq), MATLAB Function13/2(SampleTime_div_Lq), MATLAB Function14/2(SampleTime_div_Lq), MATLAB Function15/2(SampleTime_div_Lq)
  x_phase_voltage_per_switching_state7/1 -> MATLAB Function8/16(x_phase_voltage_per_switching_state)
  q_phase_voltage_per_switching_state/1 -> MATLAB Function15/15(q_phase_voltage_per_switching_state)
  MATLAB Function15/1(J) -> J/1
  d_phase_voltage_per_switching_state5/1 -> MATLAB Function10/14(d_phase_voltage_per_switching_state)
  MATLAB Function10/1(J) -> J5/1
  y_phase_voltage_per_switching_state5/1 -> MATLAB Function10/17(y_phase_voltage_per_switching_state)
  q_phase_voltage_per_switching_state6/1 -> MATLAB Function9/15(q_phase_voltage_per_switching_state)
  y_phase_voltage_per_switching_state6/1 -> MATLAB Function9/17(y_phase_voltage_per_switching_state)
  x_phase_voltage_per_switching_state6/1 -> MATLAB Function9/16(x_phase_voltage_per_switching_state)
  MATLAB Function9/1(J) -> J6/1
  MATLAB Function12/1(J) -> J3/1
  q_phase_voltage_per_switching_state7/1 -> MATLAB Function8/15(q_phase_voltage_per_switching_state)
  y_phase_voltage_per_switching_state3/1 -> MATLAB Function12/17(y_phase_voltage_per_switching_state)
  q_phase_voltage_per_switching_state3/1 -> MATLAB Function12/15(q_phase_voltage_per_switching_state)
  ix_ref15/1 -> MATLAB Function8/20(ix_ref), MATLAB Function9/20(ix_ref), MATLAB Function10/20(ix_ref), MATLAB Function11/20(ix_ref), MATLAB Function12/20(ix_ref), MATLAB Function13/20(ix_ref), MATLAB Function14/20(ix_ref), MATLAB Function15/20(ix_ref)
  iq_ref15/1 -> MATLAB Function8/19(iq_ref), MATLAB Function9/19(iq_ref), MATLAB Function10/19(iq_ref), MATLAB Function11/19(iq_ref), MATLAB Function12/19(iq_ref), MATLAB Function13/19(iq_ref), MATLAB Function14/19(iq_ref), MATLAB Function15/19(iq_ref)
  id_ref15/1 -> MATLAB Function8/18(id_ref), MATLAB Function9/18(id_ref), MATLAB Function10/18(id_ref), MATLAB Function11/18(id_ref), MATLAB Function12/18(id_ref), MATLAB Function13/18(id_ref), MATLAB Function14/18(id_ref), MATLAB Function15/18(id_ref)
  Ld15/1 -> MATLAB Function8/12(Ld), MATLAB Function9/12(Ld), MATLAB Function10/12(Ld), MATLAB Function11/12(Ld), MATLAB Function12/12(Ld), MATLAB Function13/12(Ld), MATLAB Function14/12(Ld), MATLAB Function15/12(Ld)
  iy_k_16/1 -> MATLAB Function8/8(iy_k_1), MATLAB Function9/8(iy_k_1), MATLAB Function10/8(iy_k_1), MATLAB Function11/8(iy_k_1), MATLAB Function12/8(iy_k_1), MATLAB Function13/8(iy_k_1), MATLAB Function14/8(iy_k_1), MATLAB Function15/8(iy_k_1)
  ix_k_16/1 -> MATLAB Function8/7(ix_k_1), MATLAB Function9/7(ix_k_1), MATLAB Function10/7(ix_k_1), MATLAB Function11/7(ix_k_1), MATLAB Function12/7(ix_k_1), MATLAB Function13/7(ix_k_1), MATLAB Function14/7(ix_k_1), MATLAB Function15/7(ix_k_1)
  iq_k_16/1 -> MATLAB Function8/6(iq_k_1), MATLAB Function9/6(iq_k_1), MATLAB Function10/6(iq_k_1), MATLAB Function11/6(iq_k_1), MATLAB Function12/6(iq_k_1), MATLAB Function13/6(iq_k_1), MATLAB Function14/6(iq_k_1), MATLAB Function15/6(iq_k_1)
  id_k_16/1 -> MATLAB Function8/5(id_k_1), MATLAB Function9/5(id_k_1), MATLAB Function10/5(id_k_1), MATLAB Function11/5(id_k_1), MATLAB Function12/5(id_k_1), MATLAB Function13/5(id_k_1), MATLAB Function14/5(id_k_1), MATLAB Function15/5(id_k_1)
